simulink model "SimulinkModel"  (R2019a)
settings: Solver=VariableStepAuto  StartTime=0.0  StopTime=160  RelTol=1e-3
values from neighbouring files (symbols this model uses):
  m1 = 2.294    [MD1.m]    (also in PlotModeShapes.m; animateFlexibleStructure.m; animateFlexibleStructureParFor.m)
  m2 = 1.941    [MD1.m]    (also in PlotModeShapes.m; animateFlexibleStructure.m; animateFlexibleStructureParFor.m)
  m3 = 1.943    [MD1.m]    (also in PlotModeShapes.m; animateFlexibleStructure.m; animateFlexibleStructureParFor.m)
  m4 = 2.732    [MD1.m]    (also in PlotModeShapes.m; animateFlexibleStructure.m; animateFlexibleStructureParFor.m)
  m5 = 0.774    [MD1.m]    (also in PlotModeShapes.m; animateFlexibleStructure.m; animateFlexibleStructureParFor.m)
  m6 = 0.774    [MD1.m]    (also in PlotModeShapes.m; animateFlexibleStructure.m; animateFlexibleStructureParFor.m)
undefined symbols (not defined in the file or in its folder): k1, k2, k3, k4, k5, k6
settings Model: Creator=JacobOesterby  LastModifiedBy=JacobOesterby

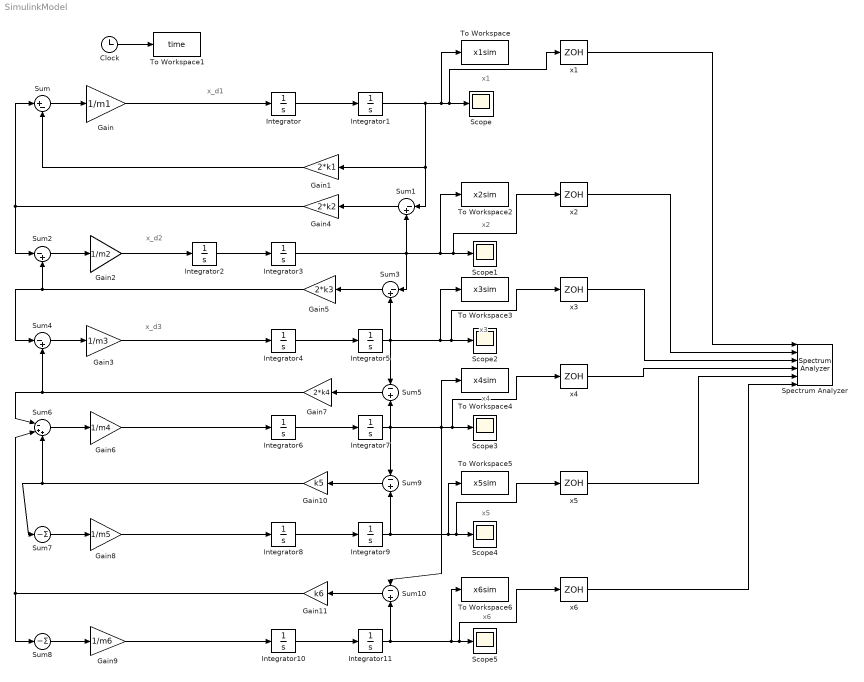
== system SimulinkModel ==
  note: x6
  note: x5
  note: x4
  note: x1
  note: x2
  note: x3
  note: x_d3
  note: x_d2
  note: x_d1
  Clock : Clock
  Gain : Gain  Gain=1/m1
  Gain1 : Gain  Gain=2*k1
  Gain10 : Gain  Gain=k5
  Gain11 : Gain  Gain=k6
  Gain2 : Gain  Gain=1/m2
  Gain3 : Gain  Gain=1/m3
  Gain4 : Gain  Gain=2*k2
  Gain5 : Gain  Gain=2*k3
  Gain6 : Gain  Gain=1/m4
  Gain7 : Gain  Gain=2*k4
  Gain8 : Gain  Gain=1/m5
  Gain9 : Gain  Gain=1/m6
  Integrator{,2..11} (11 alike) : Integrator
  Integrator1 : Integrator  InitialCondition=3
  Scope{,1..5} (6 alike) : Scope
  Spectrum Analyzer : SpectrumAnalyzer  NumInputPorts=6
  Sum : Sum  Inputs=|+-
  Sum{1..4} (4 alike) : Sum  Inputs=|-+
  Sum10 : Sum  Inputs=-+
  Sum5 : Sum  Inputs=-+
  Sum6 : Sum  Inputs=|-++
  Sum7 : Sum  Inputs=-
  Sum8 : Sum  Inputs=-
  Sum9 : Sum  Inputs=-+
  To Workspace : ToWorkspace  VariableName=x1sim  SampleTime=-1
  To Workspace1 : ToWorkspace  VariableName=time  SampleTime=0.001
  To Workspace2 : ToWorkspace  VariableName=x2sim  SampleTime=-1
  To Workspace3 : ToWorkspace  VariableName=x3sim  SampleTime=-1
  To Workspace4 : ToWorkspace  VariableName=x4sim  SampleTime=-1
  To Workspace5 : ToWorkspace  VariableName=x5sim  SampleTime=-1
  To Workspace6 : ToWorkspace  VariableName=x6sim  SampleTime=-1
  x{1..6} (6 alike) : ZeroOrderHold  SampleTime=0.001
  wires:
  Clock/1 -> To Workspace1/1
  Gain/1 -> Integrator/1
  Integrator/1 -> Integrator1/1
  Gain1/1 -> Sum/2
  Sum/1 -> Gain/1
  Gain2/1 -> Integrator2/1
  Integrator2/1 -> Integrator3/1
  Integrator3/1 -> Sum1/2, To Workspace2/1, x2/1, Scope1/1, Sum3/1
  Sum1/1 -> Gain4/1
  Gain4/1 -> Sum2/1, Sum/1
  Sum2/1 -> Gain2/1
  Gain3/1 -> Integrator4/1
  Integrator4/1 -> Integrator5/1
  Integrator5/1 -> Sum5/1, To Workspace3/1, x3/1, Scope2/1, Sum3/2
  Sum4/1 -> Gain3/1
  Sum3/1 -> Gain5/1
  Gain5/1 -> Sum4/1, Sum2/2
  Sum6/1 -> Gain6/1
  Gain6/1 -> Integrator6/1
  Integrator6/1 -> Integrator7/1
  Integrator7/1 -> Sum9/1, To Workspace4/1, x4/1, Scope3/1, Sum10/1, Sum5/2
  Sum5/1 -> Gain7/1
  Gain7/1 -> Sum6/1, Sum4/2
  Sum7/1 -> Gain8/1
  Gain8/1 -> Integrator8/1
  Integrator8/1 -> Integrator9/1
  Integrator9/1 -> To Workspace5/1, x5/1, Scope4/1, Sum9/2
  Sum8/1 -> Gain9/1
  Gain9/1 -> Integrator10/1
  Integrator10/1 -> Integrator11/1
  Integrator11/1 -> To Workspace6/1, x6/1, Scope5/1, Sum10/2
  Sum9/1 -> Gain10/1
  Gain10/1 -> Sum7/1, Sum6/3
  Sum10/1 -> Gain11/1
  Gain11/1 -> Sum8/1, Sum6/2
  Integrator1/1 -> To Workspace/1, x1/1, Scope/1, Gain1/1, Sum1/1
  x1/1 -> Spectrum Analyzer/1
  x2/1 -> Spectrum Analyzer/2
  x3/1 -> Spectrum Analyzer/3
  x4/1 -> Spectrum Analyzer/4
  x5/1 -> Spectrum Analyzer/5
  x6/1 -> Spectrum Analyzer/6
